simulink model "Grid_Forming_Droop_Control"  (R2022b)
settings: Solver=VariableStepAuto  StartTime=0.0  StopTime=50  RelTol=1e-3
values from neighbouring files (symbols this model uses):
  C_dc = 0.008*(n)    (= 1.6)    [Grid_Forming_Droop_Control_Code.m]
  C_f = n*300*10^-6    (= 0.06)    [Grid_Forming_Droop_Control_Code.m]
  f_0 = 50    [Grid_Forming_Droop_Control_Code.m]
  i_ll = 5*-1.15*(S_b/Vdc_n)-i_loss_dc    [Grid_Forming_Droop_Control_Code.m]
  i_ul = 5*1.15*(S_b/Vdc_n)+i_loss_dc    [Grid_Forming_Droop_Control_Code.m]
  k_dc = eta_1/(Vdc_n*m_p)    [Grid_Forming_Droop_Control_Code.m]
  K_p = (1/Vdc_n)    [Grid_Forming_Droop_Control_Code.m]
  K_r = 1/R_dc    [Grid_Forming_Droop_Control_Code.m]
  Kff_i = 1    [Grid_Forming_Droop_Control_Code.m]
  Kff_v = 1    [Grid_Forming_Droop_Control_Code.m]
  Ki_i = (1/n)*1.19    (= 0.00595)    [Grid_Forming_Droop_Control_Code.m]
  Ki_v = (n)*1.161022    (= 232.2044)    [Grid_Forming_Droop_Control_Code.m]
  ki_v_ac = 2*0.25    (= 0.5)    [Grid_Forming_Droop_Control_Code.m]
  Kp_i = 0.738891    [Grid_Forming_Droop_Control_Code.m]
  Kp_v = 0.52    [Grid_Forming_Droop_Control_Code.m]
  kp_v_ac = 0.001    [Grid_Forming_Droop_Control_Code.m]
  L_f = (1/n)*200*10^-6    (= 1e-06)    [Grid_Forming_Droop_Control_Code.m]
  m_p = (2*pi*(f_0*0.01))/(S_b)    [Grid_Forming_Droop_Control_Code.m]
  n = 200    [Grid_Forming_Droop_Control_Code.m]
  R_dc = (Vdc_n/(0.05*(S_b)/Vdc_n))    [Grid_Forming_Droop_Control_Code.m]
  R_f = 0.001/n    (= 5e-06)    [Grid_Forming_Droop_Control_Code.m]
  S_b = 10*(10^6)    (= 10000000)    [Grid_Forming_Droop_Control_Code.m]
  T_en = T_load-0.5    (= 24.5)    [Grid_Forming_Droop_Control_Code.m]
  T_s = 1e-4    (= 0.0001)    [Grid_Forming_Droop_Control_Code.m]
  tau_dc = 0.05    [Grid_Forming_Droop_Control_Code.m]
  V_m = sqrt(2/3)*V1_rms    [Grid_Forming_Droop_Control_Code.m]
  Vdc_n = 3*V_m    [Grid_Forming_Droop_Control_Code.m]
  Vg = 1000    [Grid_Forming_Droop_Control_Code.m]
  w_b = 2*pi*f_b    (= 314.159265359)    [Grid_Forming_Droop_Control_Code.m]
  w_f = 2*pi*0.1*f_b    (= 31.4159265359)    [Grid_Forming_Droop_Control_Code.m]
undefined symbols (not defined in the file or in its folder): i_dc
libraries: spsSeriesRLCBranchLib x8, spsVoltageMeasurementLib x8, spsCurrentMeasurementLib x7, spsabctodq0Lib x7, spsGroundLib x3, spsFirstOrderFilterLib x2, cstblocks x1, spsControlledCurrentSourceLib x1, slpidlib x1, spsThreePhaseSourceLib x1, spsUniversalBridgeLib x1, spsdq0toabcLib x1
settings Model: Creator=alper.cakiroglu  LastModifiedBy=alper.cakiroglu

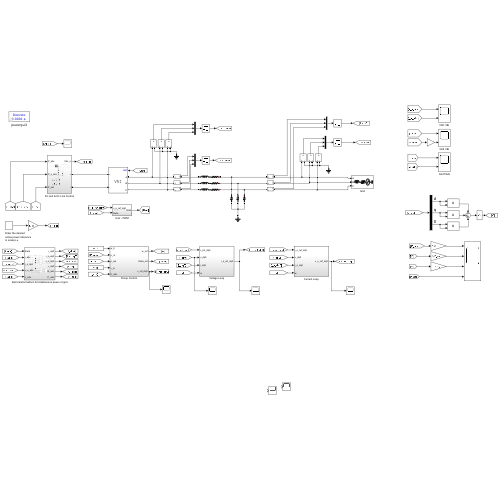
[thumbnail: Simulink's stored preview of the top-level diagram]
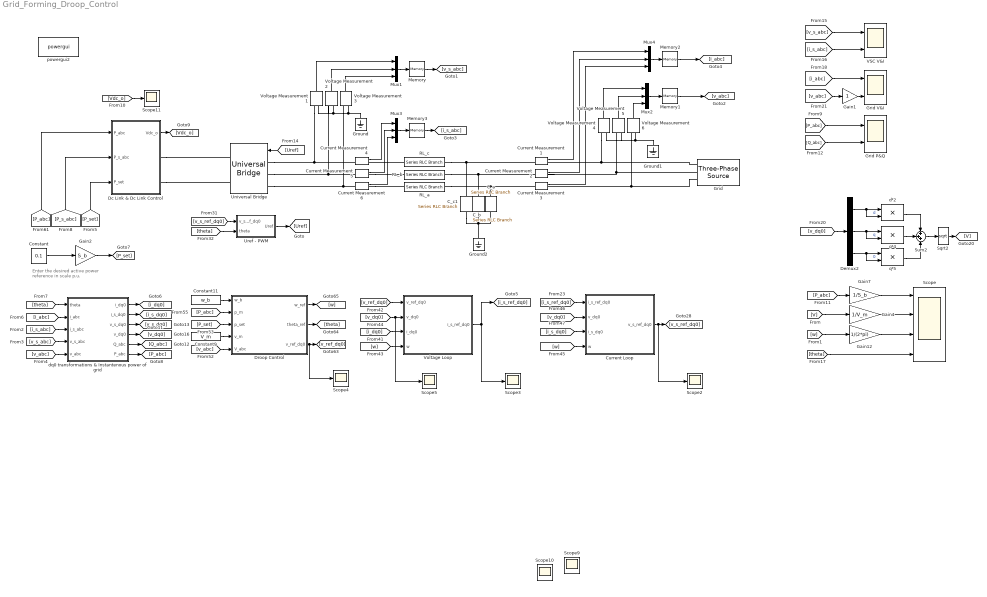
== system Grid_Forming_Droop_Control ==
  note: Enter the desired active power reference
      | in scale p.u.
  C_a : spsSeriesRLCBranchLib/Series RLC Branch  LConnTagsString=__new0  RConnTagsString=__new0  BranchType=C  Resistance=1  Inductance=1e-3  SetiL0=off  InitialCurrent=0  Capacitance=C_f  Setx0=off  InitialVoltage=165  Measurements=None
  C_b : spsSeriesRLCBranchLib/Series RLC Branch  LConnTagsString=__new0  RConnTagsString=__new0  BranchType=C  Resistance=1  Inductance=1e-3  SetiL0=off  InitialCurrent=0  Capacitance=C_f  Setx0=off  InitialVoltage=165  Measurements=None
  C_c1 : spsSeriesRLCBranchLib/Series RLC Branch  LConnTagsString=__new0  RConnTagsString=__new0  BranchType=C  Resistance=1  Inductance=1e-3  SetiL0=off  InitialCurrent=0  Capacitance=C_f  Setx0=off  InitialVoltage=165  Measurements=None
  Constant : Constant  Value=0.1
  Constant11 : Constant  Value=w_b
  Constant9 : Constant  Value=V_m
  Current Loop : Subsystem
  Current Measurement{1..6} (6 alike) : spsCurrentMeasurementLib/Current Measurement  PhasorSimulation=off  OutputType=Complex  PSBequivalent=0
  Dc Link & Dc Link Control : Subsystem
  Demux2 : Demux  Outputs=3
  Droop Control : Subsystem
  Gain1 : Gain
  Gain12 : Gain  Gain=1/(2*pi)
  Gain2 : Gain  Gain=S_b
  Gain4 : Gain  Gain=1/V_m
  Gain7 : Gain  Gain=1/S_b
  Grid : spsThreePhaseSourceLib/Three-Phase Source  InternalConnection=Yg  VoltagePhases=off  Voltage=Vg  PhaseAngle=0  Voltage_phases=[25e3 25e3 25e3]/sqrt(3)  PhaseAngles_phases=[0 -120 +120]  Frequency=f_0  NonIdealSource=on  SpecifyImpedance=on  Resistance=0.8929  Inductance=16.58e-3  ShortCircuitLevel=S_b  BaseVoltage=Vg  XRratio=10  BusType=swing  Pref=10e3  Qref=0  Prefabc=[10e3, 10e3, 10e3]  Qrefabc=[0, 0, 0]  Qmin=-inf  Qmax=inf
  Grid P&Q : Scope  NumInputPorts=2
  Grid V&I : Scope  NumInputPorts=2
  Ground : spsGroundLib/Ground  LConnTagsString=a
  Ground1 : spsGroundLib/Ground  LConnTagsString=a
  Ground2 : spsGroundLib/Ground  LConnTagsString=a
  Memory{,1..3} (4 alike) : Memory
  Mux{1..4} (4 alike) : Mux  Inputs=3
  RL_a : spsSeriesRLCBranchLib/Series RLC Branch  LConnTagsString=__new0  RConnTagsString=__new0  BranchType=RL  Resistance=R_f  Inductance=L_f  SetiL0=off  InitialCurrent=0  Capacitance=1e-6  Setx0=off  InitialVoltage=0  Measurements=Branch voltage and current
  RL_b : spsSeriesRLCBranchLib/Series RLC Branch  LConnTagsString=__new0  RConnTagsString=__new0  BranchType=RL  Resistance=R_f  Inductance=L_f  SetiL0=off  InitialCurrent=0  Capacitance=1e-6  Setx0=off  InitialVoltage=0  Measurements=None
  RL_c : spsSeriesRLCBranchLib/Series RLC Branch  LConnTagsString=__new0  RConnTagsString=__new0  BranchType=RL  Resistance=R_f  Inductance=L_f  SetiL0=off  InitialCurrent=0  Capacitance=1e-6  Setx0=off  InitialVoltage=0  Measurements=None
  Scope : Scope  NumInputPorts=4
  Scope{2..5,9..11} (7 alike) : Scope
  Sqrt2 : Sqrt
  Sum2 : Sum  Inputs=+++  InputSameDT=on  SaturateOnIntegerOverflow=on  OutDataTypeStr=Inherit: Same as first input
  Universal Bridge : spsUniversalBridgeLib/Universal Bridge  Arms=3  SnubberResistance=1e5  SnubberCapacitance=inf  Device=Average-model based VSC  Ron=1e-3  Lon=0  ForwardVoltages="[  0  0  ]"  ForwardVoltage=0  GTOparameters=[ 10e-6 , 20e-6 ]  IGBTparameters=[ 1e-6 , 2e-6 ]  Measurements=None  Measurements_2=None  converterType=Rectifier
  Uref - PWM : Subsystem
  VSC V&I : Scope  NumInputPorts=2
  Voltage Loop : Subsystem
  Voltage Measurement{1..6} (6 alike) : spsVoltageMeasurementLib/Voltage Measurement  PhasorSimulation=off  OutputType=Complex  PSBequivalent=0
  dq0 transformations & Instantenous power of grid : Subsystem
  d²2 : Product  InputSameDT=on  RndMeth=Zero  SaturateOnIntegerOverflow=on  OutDataTypeStr=Inherit: Same as first input
  powergui2 : sps_lib/powergui  Priority=1  SimulationMode=Discrete  SampleTime=T_s  frequency=50  Iterations=50  frequencyindice=0  Pbase=100e6  ErrMax=0.0001  UnitsV=kV  UnitsW=MW  buscounter=0  FunctionMessages=off  echomessages=off  EnableUseOfTLC=off  CurrentSourceSwitches=off  DisableSnubberDevices=off  DisableRonSwitches=off  DisableVfSwitches=off  DisplayEquations=off  AutomaticDiscreteSolvers=off  SolverType=Tustin/Backward Euler (TBE)  Interpol=off  ExternalGateDelay=off  methode=off  Ts=100  x0status=blocks  SPID=off  SwTol=0  HookPort=off  NonlinearTolerance=1e-4  nMaxIteration=100  ContinueOnMaxIteration=off  RestoreLinks=warning  ResistiveCurrentMeasurement=off  Frange=[0:2:500]  Ylog=off  Xlog=on  ShowGrid=off  save=off  variable=ZData  structure=0  ZoomFFT=off  StartTime=0.0  cycles=1  DisplayStyle=1  fundamental=60  FreqAxis=off  MaxFrequency=1000  frequencyindicesteady=1  RmsSteady=1  display=off
  q²4 : Product  InputSameDT=on  RndMeth=Zero  SaturateOnIntegerOverflow=on  OutDataTypeStr=Inherit: Same as first input
  q²5 : Product  InputSameDT=on  RndMeth=Zero  SaturateOnIntegerOverflow=on  OutDataTypeStr=Inherit: Same as first input
  wires:
  Voltage Measurement2/1 -> Mux1/2
  Voltage Measurement1/1 -> Mux1/1
  Voltage Measurement3/1 -> Mux1/3
  Memory/1 -> [v_s_abc]
  Mux1/1 -> Memory/1
  Memory1/1 -> [v_abc]
  Voltage Measurement6/1 -> Mux2/3
  Voltage Measurement4/1 -> Mux2/1
  Voltage Measurement5/1 -> Mux2/2
  Mux2/1 -> Memory1/1
  Mux3/1 -> Memory3/1
  Memory3/1 -> [i_s_abc]
  Current Measurement4/1 -> Mux3/1
  Current Measurement5/1 -> Mux3/2
  Current Measurement6/1 -> Mux3/3
  Memory2/1 -> [i_abc]
  Mux4/1 -> Memory2/1
  Current Measurement1/1 -> Mux4/1
  Current Measurement2/1 -> Mux4/2
  Current Measurement3/1 -> Mux4/3
  [v_dq0] -> Demux2/1
  Gain12/1 -> Scope/3
  [P_abc] -> Gain7/1
  Demux2/3 -> q²5/1, q²5/2  "0"
  Demux2/2 -> q²4/1, q²4/2  "q"
  q²5/1 -> Sum2/3
  Sum2/1 -> Sqrt2/1
  d²2/1 -> Sum2/1
  Constant/1 -> Gain2/1
  Sqrt2/1 -> [V]
  Demux2/1 -> d²2/1, d²2/2  "d"
  [w] -> Gain12/1
  [theta] -> Scope/4
  Gain4/1 -> Scope/2
  q²4/1 -> Sum2/2
  Gain2/1 -> [P_set]
  Gain7/1 -> Scope/1
  [V] -> Gain4/1
  [w] -> Voltage Loop/4(w)
  Droop Control/3(v_ref_dq0) -> Scope4/1, [v_ref_dq0]
  [v_dq0] -> Current Loop/2(v_dq0)
  Droop Control/1(w_ref) -> [w]
  Current Loop/1(v_s_ref_dq0) -> Scope2/1, [v_s_ref_dq0]
  Constant11/1 -> Droop Control/1(w_b)
  Voltage Loop/1(i_s_ref_dq0) -> Scope3/1, [i_s_ref_dq0]
  [w] -> Current Loop/4(w)
  [v_abc] -> Droop Control/5(V_abc)
  [v_ref_dq0] -> Voltage Loop/1(v_ref_dq0)
  [i_dq0] -> Voltage Loop/3(i_dq0)
  [i_s_dq0] -> Current Loop/3(i_s_dq0)
  [v_dq0] -> Scope5/1, Voltage Loop/2(v_dq0)
  Droop Control/2(theta_ref) -> [theta]
  [P_set] -> Droop Control/3(p_set)
  [P_abc] -> Droop Control/2(p_m)
  [Vdc_o] -> Scope11/1
  Constant9/1 -> Droop Control/4(v_m)
  Dc Link & Dc Link Control/1(Vdc_o) -> [Vdc_o]
  [P_abc] -> Dc Link & Dc Link Control/1(P_abc)
  [P_s_abc] -> Dc Link & Dc Link Control/2(P_s_abc)
  [P_set] -> Dc Link & Dc Link Control/3(P_set)
  [Uref] -> Universal Bridge/1
  [v_s_abc] -> VSC V&I/1
  [i_s_abc] -> VSC V&I/2
  Uref - PWM/1(Uref) -> [Uref]
  [v_s_ref_dq0] -> Uref - PWM/1(v_s_ref_dq0)
  [theta] -> Uref - PWM/2(theta)
  [i_abc] -> Grid V&I/1
  [v_abc] -> Gain1/1
  Gain1/1 -> Grid V&I/2
  [i_abc] -> dq0 transformations & Instantenous power of grid/2(i_abc)
  [i_s_abc] -> dq0 transformations & Instantenous power of grid/3(i_s_abc)
  [v_s_abc] -> dq0 transformations & Instantenous power of grid/4(v_s_abc)
  [v_abc] -> dq0 transformations & Instantenous power of grid/5(v_abc)
  dq0 transformations & Instantenous power of grid/1(i_dq0) -> [i_dq0]
  dq0 transformations & Instantenous power of grid/2(i_s_dq0) -> [i_s_dq0]
  dq0 transformations & Instantenous power of grid/3(v_s_dq0) -> [v_s_dq0]
  dq0 transformations & Instantenous power of grid/4(v_dq0) -> [v_dq0]
  dq0 transformations & Instantenous power of grid/5(Q_abc) -> [Q_abc]
  dq0 transformations & Instantenous power of grid/6(P_abc) -> [P_abc]
  [theta] -> dq0 transformations & Instantenous power of grid/1(theta)
  [i_s_ref_dq0] -> Current Loop/1(i_s_ref_dq0)
  [Q_abc] -> Grid P&Q/2
  [P_abc] -> Grid P&Q/1
  connections:
  Universal Bridge/LConn1 -- Voltage Measurement1/LConn1 -- Current Measurement4/LConn1
  Universal Bridge/LConn2 -- Voltage Measurement2/LConn1 -- Current Measurement5/LConn1
  Universal Bridge/LConn3 -- Voltage Measurement3/LConn1 -- Current Measurement6/LConn1
  Voltage Measurement1/LConn2 -- Voltage Measurement2/LConn2 -- Voltage Measurement3/LConn2 -- Ground/LConn1
  RL_c/RConn1 -- Current Measurement4/RConn1
  Current Measurement5/RConn1 -- RL_b/RConn1
  Current Measurement6/RConn1 -- RL_a/RConn1
  Ground2/LConn1 -- C_c1/RConn1 -- C_a/RConn1 -- C_b/RConn1
  RL_c/LConn1 -- C_c1/LConn1 -- Current Measurement1/LConn1
  RL_b/LConn1 -- C_b/LConn1 -- Current Measurement2/LConn1
  RL_a/LConn1 -- C_a/LConn1 -- Current Measurement3/LConn1
  Grid/RConn1 -- Voltage Measurement4/LConn1 -- Current Measurement1/RConn1
  Current Measurement2/RConn1 -- Voltage Measurement5/LConn1 -- Grid/RConn2
  Grid/RConn3 -- Voltage Measurement6/LConn1 -- Current Measurement3/RConn1
  Voltage Measurement6/LConn2 -- Voltage Measurement4/LConn2 -- Voltage Measurement5/LConn2 -- Ground1/LConn1
  Dc Link & Dc Link Control/RConn2 -- Universal Bridge/RConn2
  Dc Link & Dc Link Control/RConn1 -- Universal Bridge/RConn1

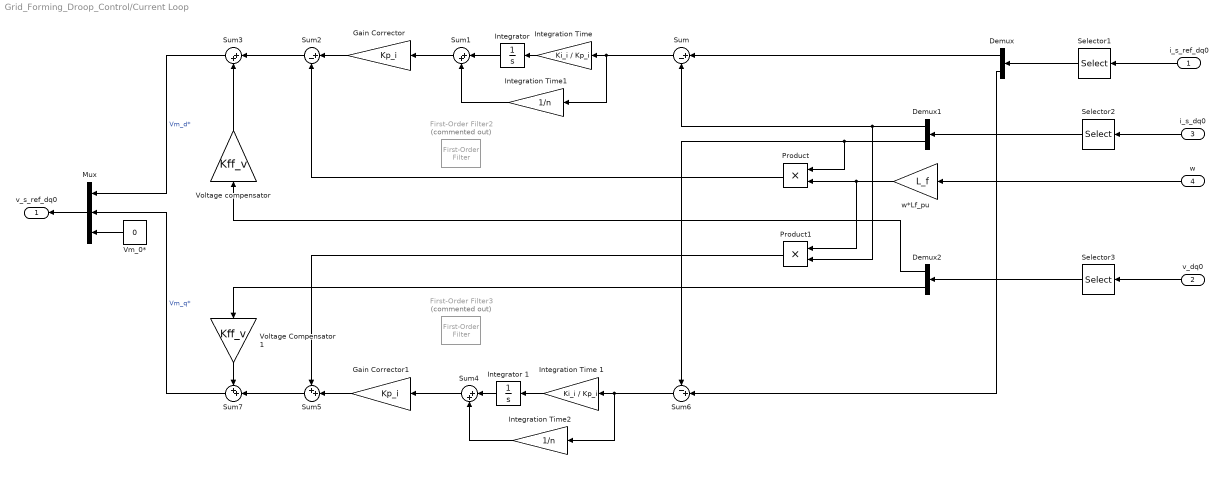
== system Grid_Forming_Droop_Control/Current Loop ==
  i_s_ref_dq0 : Inport
  v_dq0 : Inport  Port=2
  i_s_dq0 : Inport  Port=3
  w : Inport  Port=4
  Demux : Demux  Outputs=2
  Demux1 : Demux  Outputs=2
  Demux2 : Demux  Outputs=2
  First-Order Filter2 : spsFirstOrderFilterLib/First-Order Filter  Commented=on  FilterType=Lowpass  Tc=25e-3  Ts=0  Initialize=on  Vac_Init=[0, 0, 50]  Vdc_Init=1  PlotResponse=off  FreqRange="[0,  200,  1]"
  First-Order Filter3 : spsFirstOrderFilterLib/First-Order Filter  Commented=on  FilterType=Lowpass  Tc=25e-3  Ts=0  Initialize=on  Vac_Init=[0, 0, 50]  Vdc_Init=0  PlotResponse=off  FreqRange="[0,  200,  1]"
  Gain Corrector : Gain  Gain=Kp_i
  Gain Corrector1 : Gain  Gain=Kp_i
  Integration Time : Gain  Gain=Ki_i / Kp_i
  Integration Time 1 : Gain  Gain=Ki_i / Kp_i
  Integration Time1 : Gain  Gain=1/n
  Integration Time2 : Gain  Gain=1/n
  Integrator : Integrator  InitialCondition=0.0001
  Integrator 1 : Integrator
  Mux : Mux  Inputs=3
  Product : Product  RndMeth=Zero
  Product1 : Product  RndMeth=Zero
  Selector1 : Selector  InputPortWidth=3  IndexOptions=Index vector (dialog)  Indices=[1 2]  OutputSizes=1
  Selector2 : Selector  InputPortWidth=3  IndexOptions=Index vector (dialog)  Indices=[1 2]  OutputSizes=1
  Selector3 : Selector  InputPortWidth=3  IndexOptions=Index vector (dialog)  Indices=[1 2]  OutputSizes=1
  Sum : Sum  Inputs=|+-
  Sum1 : Sum  Inputs=|++
  Sum2 : Sum  Inputs=|+-
  Sum3 : Sum  Inputs=|++
  Sum4 : Sum  Inputs=|++
  Sum5 : Sum  Inputs=++|
  Sum6 : Sum  Inputs=-+|
  Sum7 : Sum  Inputs=++|
  Vm_0* : Constant  Value=0
  Voltage Compensator 1 : Gain  Gain=Kff_v
  Voltage compensator : Gain  Gain=Kff_v
  w*Lf_pu : Gain  Gain=L_f
  v_s_ref_dq0 : Outport  VectorParamsAs1DForOutWhenUnconnected=off
  wires:
  Sum/1 -> Integration Time/1, Integration Time1/1
  Integration Time 1/1 -> Integrator 1/1
  Integration Time/1 -> Integrator/1
  Sum5/1 -> Sum7/2
  Sum6/1 -> Integration Time 1/1, Integration Time2/1
  Demux/1 -> Sum/1
  Sum3/1 -> Mux/1  "Vm_d*"
  Sum7/1 -> Mux/2  "Vm_q*"
  Demux2/2 -> Voltage Compensator 1/1
  Voltage Compensator 1/1 -> Sum7/1
  Product/1 -> Sum2/2
  w*Lf_pu/1 -> Product1/1, Product/2
  i_s_ref_dq0/1 -> Selector1/1
  v_dq0/1 -> Selector3/1
  Integrator 1/1 -> Sum4/1
  Voltage compensator/1 -> Sum3/2
  Sum1/1 -> Gain Corrector/1
  Sum2/1 -> Sum3/1
  Sum4/1 -> Gain Corrector1/1
  Demux/2 -> Sum6/2
  Selector1/1 -> Demux/1
  Gain Corrector/1 -> Sum2/1
  w/1 -> w*Lf_pu/1
  Mux/1 -> v_s_ref_dq0/1
  Selector2/1 -> Demux1/1
  i_s_dq0/1 -> Selector2/1
  Selector3/1 -> Demux2/1
  Demux1/2 -> Product/1, Sum6/1
  Vm_0*/1 -> Mux/3
  Integrator/1 -> Sum1/1
  Demux1/1 -> Product1/2, Sum/2
  Demux2/1 -> Voltage compensator/1
  Product1/1 -> Sum5/1
  Gain Corrector1/1 -> Sum5/2
  Integration Time1/1 -> Sum1/2
  Integration Time2/1 -> Sum4/2

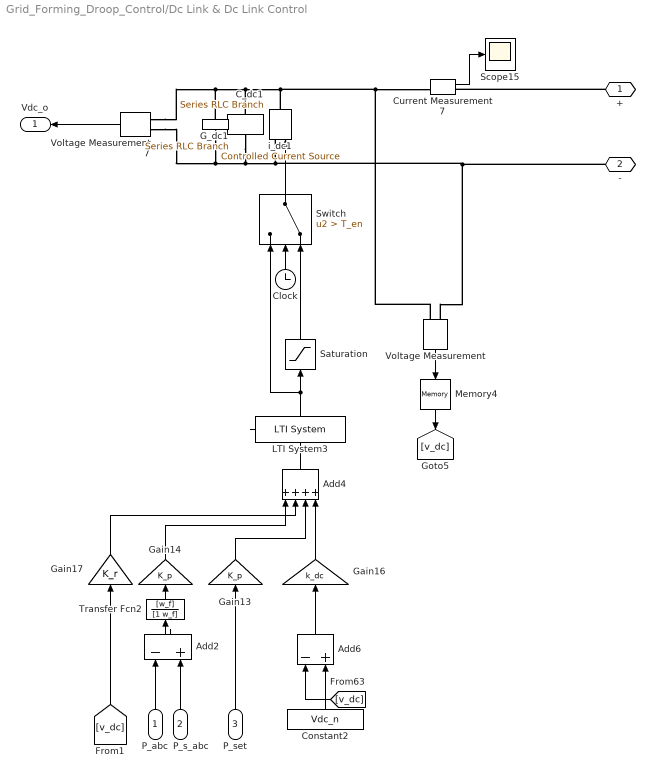
== system Grid_Forming_Droop_Control/Dc Link & Dc Link Control ==
  P_abc : Inport
  P_s_abc : Inport  Port=2
  P_set : Inport  Port=3
  Add2 : Sum  Inputs=+-
  Add4 : Sum  Inputs=++++
  Add6 : Sum  Inputs=+-
  C_dc1 : spsSeriesRLCBranchLib/Series RLC Branch  LConnTagsString=__new0  RConnTagsString=__new0  BranchType=C  Resistance=1  Inductance=1e-3  SetiL0=off  InitialCurrent=0  Capacitance=C_dc  Setx0=off  InitialVoltage=Vdc_n  Measurements=None
  Clock : Clock
  Constant2 : Constant  Value=Vdc_n
  Current Measurement7 : spsCurrentMeasurementLib/Current Measurement  PhasorSimulation=off  OutputType=Complex  PSBequivalent=0
  G_dc1 : spsSeriesRLCBranchLib/Series RLC Branch  LConnTagsString=__new0  RConnTagsString=__new0  BranchType=R  Resistance=R_dc  Inductance=1e-3  SetiL0=off  InitialCurrent=0  Capacitance=1e-6  Setx0=off  InitialVoltage=0  Measurements=None
  Gain13 : Gain  Gain=K_p
  Gain14 : Gain  Gain=K_p
  Gain16 : Gain  Gain=k_dc
  Gain17 : Gain  Gain=K_r
  LTI System3 : cstblocks/LTI System  sys=tf(1,[tau_dc 1])  IC=[]
  Memory4 : Memory
  Saturation : Saturate  UpperLimit=i_ul  LowerLimit=i_ll
  Scope15 : Scope
  Switch : Switch  Criteria=u2 > Threshold  Threshold=T_en  SaturateOnIntegerOverflow=off  InputSameDT=off
  Transfer Fcn2 : TransferFcn  Numerator=[w_f]  Denominator=[1 w_f]
  Voltage Measurement : spsVoltageMeasurementLib/Voltage Measurement  PhasorSimulation=off  OutputType=Complex  PSBequivalent=0
  Voltage Measurement7 : spsVoltageMeasurementLib/Voltage Measurement  PhasorSimulation=off  OutputType=Complex  PSBequivalent=0
  i_dc1 : spsControlledCurrentSourceLib/Controlled Current Source  Initialize=off  Source_Type=DC  Amplitude=i_dc  Phase=0  Frequency=0  Measurements=None
  + : PMIOPort  Side=Right
  - : PMIOPort  Port=2  Side=Right
  Vdc_o : Outport
  wires:
  Clock/1 -> Switch/2
  Add2/1 -> Transfer Fcn2/1
  Gain16/1 -> Add4/1
  Current Measurement7/1 -> Scope15/1
  Switch/1 -> i_dc1/1
  Saturation/1 -> Switch/1
  Transfer Fcn2/1 -> Gain14/1
  Gain17/1 -> Add4/3
  Voltage Measurement/1 -> Memory4/1
  Add6/1 -> Gain16/1
  LTI System3/1 -> Switch/3, Saturation/1
  Memory4/1 -> [v_dc]
  Gain14/1 -> Add4/4
  Constant2/1 -> Add6/1
  [v_dc] -> Add6/2
  Add4/1 -> LTI System3/1
  P_s_abc/1 -> Add2/1
  Gain13/1 -> Add4/2
  P_set/1 -> Gain13/1
  Voltage Measurement7/1 -> Vdc_o/1
  P_abc/1 -> Add2/2
  [v_dc] -> Gain17/1
  connections:
  +/RConn1 -- Current Measurement7/RConn1
  Voltage Measurement/LConn1 -- Current Measurement7/LConn1 -- G_dc1/LConn1 -- Voltage Measurement7/LConn1 -- C_dc1/LConn1 -- i_dc1/RConn1
  i_dc1/LConn1 -- -/RConn1 -- Voltage Measurement/LConn2 -- G_dc1/RConn1 -- Voltage Measurement7/LConn2 -- C_dc1/RConn1

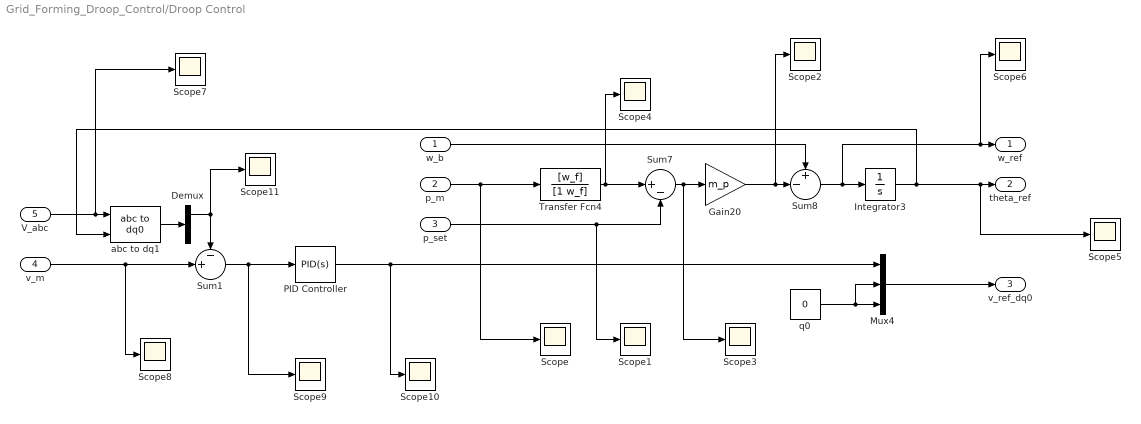
== system Grid_Forming_Droop_Control/Droop Control ==
  w_b : Inport
  p_m : Inport  Port=2
  p_set : Inport  Port=3
  v_m : Inport  Port=4
  V_abc : Inport  Port=5
  Demux : Demux  Outputs=3
  Gain20 : Gain  Gain=m_p
  Integrator3 : Integrator
  Mux4 : Mux  Inputs=3
  PID Controller : slpidlib/PID Controller  Controller=PID  Form=Parallel  TimeDomain=Continuous-time  UseExternalTs=off  SampleTime=-1  IntegratorMethod=Forward Euler  FilterMethod=Forward Euler  ControllerParametersSource=internal  P=kp_v_ac  I=ki_v_ac  UseKiTs=off  D=0  N=100  UseFilter=on  TunerSelectOption=Transfer Function Based (PID Tuner App)  InitialConditionSource=internal  InitialConditionForIntegrator=0  InitialConditionForFilter=0  DifferentiatorICPrevScaledInput=0  ExternalReset=none  TrackingMode=off  Kt=1  LimitOutput=off  SatLimitsSource=internal  UpperSaturationLimit=inf  LowerSaturationLimit=-inf  LinearizeAsGain=on  AntiWindupMode=none  Kb=1  LimitIntegrator=off  UpperIntegratorSaturationLimit=inf  LowerIntegratorSaturationLimit=-inf  POutMin=[]  POutMax=[]  IOutMin=[]  IOutMax=[]  DOutMin=[]  DOutMax=[]  NOutMin=[]  NOutMax=[]  SumOutMin=[]  SumOutMax=[]  SaturationOutMin=[]  SaturationOutMax=[]  PParamMin=[]  PParamMax=[]  IParamMin=[]  IParamMax=[]  DParamMin=[]  DParamMax=[]  NParamMin=[]  NParamMax=[]  KbParamMin=[]  KbParamMax=[]  KtParamMin=[]  KtParamMax=[]  KbOutMin=[]  KbOutMax=[]  KtOutMin=[]  KtOutMax=[]  IntegratorOutMin=[]  IntegratorOutMax=[]  FilterOutMin=[]  FilterOutMax=[]  SumI1OutMin=[]  SumI1OutMax=[]  SumI2OutMin=[]  SumI2OutMax=[]  SumI3OutMin=[]  SumI3OutMax=[]  SumI4OutMin=[]  SumI4OutMax=[]  SumDOutMin=[]  SumDOutMax=[]  DifferentiatorOutMin=[]  DifferentiatorOutMax=[]  FilterDiffOutCoefMin=[]  FilterDiffOutCoefMax=[]  ReciprocalOutMin=[]  ReciprocalOutMax=[]  SumDenOutMin=[]  SumDenOutMax=[]  SumNumOutMin=[]  SumNumOutMax=[]  DivideOutMin=[]  DivideOutMax=[]  UdiffTsProdOutMin=[]  UdiffTsProdOutMax=[]  NTsProdOutMin=[]  NTsProdOutMax=[]  UintegralTsProdOutMin=[]  UintegralTsProdOutMax=[]  UngainTsProdOutMin=[]  UngainTsProdOutMax=[]  ClampingZeroOutDataTypeStr=Inherit: Inherit via back propagation  ClampingZeroOutMin=[]  ClampingZeroOutMax=[]  FilterDenConstantOutDataTypeStr=Inherit: Inherit via back propagation  FilterDenConstantOutMin=[]  FilterDenConstantOutMax=[]  PCopyOutDataTypeStr=Inherit: Inherit via back propagation  PCopyOutMin=[]  PCopyOutMax=[]  NCopyOutDataTypeStr=Inherit: Inherit via back propagation  NCopyOutMin=[]  NCopyOutMax=[]  IntegratorContinuousStateAttributes=''  IntegratorStateMustResolveToSignalObject=off  IntegratorRTWStateStorageClass=Auto  FilterContinuousStateAttributes=''  FilterStateMustResolveToSignalObject=off  FilterRTWStateStorageClass=Auto  ParallelPVariant=InternalParameters  IdealPVariant=Disabled  IVariant=InternalParameters  DVariant=InternalParameters  IntegratorVariant=Continuous  SatVariant=Disabled  AWVariant=Passthrough  PCopyVariant=Disabled  TRVariant=Disabled  FdbkBlocksVariant=Forward  IdealPFdbkVariant=Disabled  SatFdbkVariant=Disabled  DerivativeFilterVariant=ContFilter  NVariant=InternalParameters  NCopyVariant=Disabled  FilterICVariant=InternalICsFilter  IntegratorICVariant=InternalICs  ExternalResetVariant=Disabled  TRSumVariant=Passthrough  SumFdbkVariant=Disabled  SumVariant=Sum_PID  TsampFilterVariant=InternalTs  TsampNgainVariant=Passthrough  TsampIntegralVariant=Passthrough  ExternalSaturationOutDataTypeStr=Inherit: Same as second input
  Scope{,1..11} (12 alike) : Scope
  Sum1 : Sum  Inputs=-+|
  Sum7 : Sum  Inputs=|+-
  Sum8 : Sum  Inputs=+-|
  Transfer Fcn4 : TransferFcn  Numerator=[w_f]  Denominator=[1 w_f]
  abc to dq1 : spsabctodq0Lib/abc to dq0  Alignment=90 degrees behind phase A axis
  q0 : Constant  Value=0
  w_ref : Outport  VectorParamsAs1DForOutWhenUnconnected=off
  theta_ref : Outport  Port=2  VectorParamsAs1DForOutWhenUnconnected=off
  v_ref_dq0 : Outport  Port=3  VectorParamsAs1DForOutWhenUnconnected=off
  wires:
  Demux/1 -> Scope11/1, Sum1/1
  abc to dq1/1 -> Demux/1
  Transfer Fcn4/1 -> Scope4/1, Sum7/1
  Mux4/1 -> v_ref_dq0/1
  q0/1 -> Mux4/3, Mux4/2
  Sum8/1 -> Integrator3/1, Scope6/1, w_ref/1
  Gain20/1 -> Scope2/1, Sum8/2
  Sum7/1 -> Scope3/1, Gain20/1
  p_m/1 -> Transfer Fcn4/1, Scope/1
  p_set/1 -> Sum7/2, Scope1/1
  w_b/1 -> Sum8/1
  V_abc/1 -> Scope7/1, abc to dq1/1
  Sum1/1 -> PID Controller/1, Scope9/1
  v_m/1 -> Scope8/1, Sum1/2
  Integrator3/1 -> abc to dq1/2, Scope5/1, theta_ref/1
  PID Controller/1 -> Scope10/1, Mux4/1

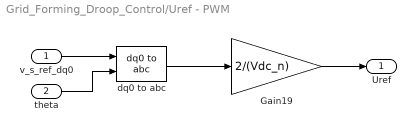
== system Grid_Forming_Droop_Control/Uref - PWM ==
  v_s_ref_dq0 : Inport
  theta : Inport  Port=2
  Gain19 : Gain  Gain=2/(Vdc_n)
  dq0 to abc : spsdq0toabcLib/dq0 to abc  Alignment=90 degrees behind phase A axis
  Uref : Outport
  wires:
  v_s_ref_dq0/1 -> dq0 to abc/1
  theta/1 -> dq0 to abc/2
  dq0 to abc/1 -> Gain19/1
  Gain19/1 -> Uref/1

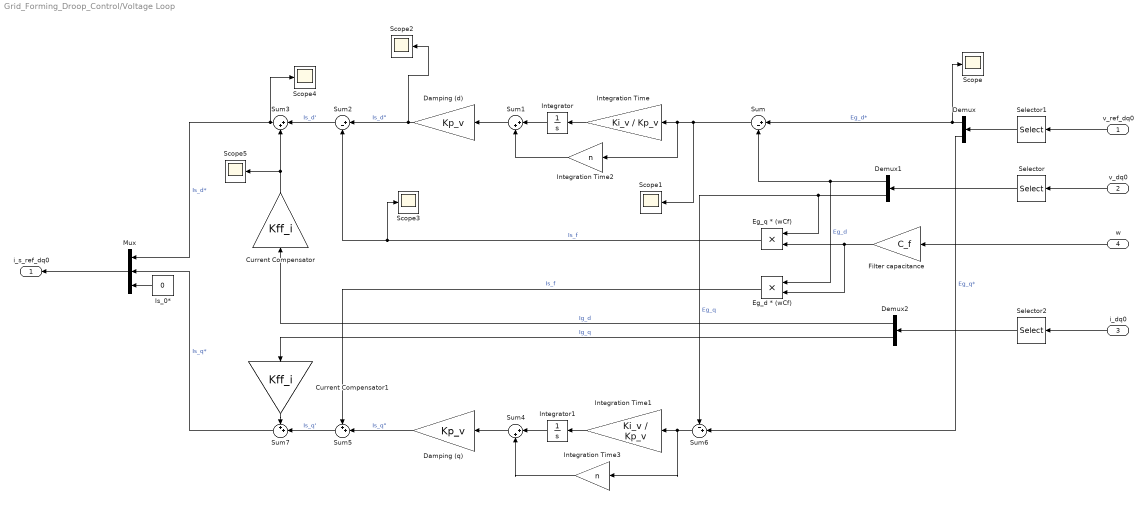
== system Grid_Forming_Droop_Control/Voltage Loop ==
  v_ref_dq0 : Inport
  v_dq0 : Inport  Port=2
  i_dq0 : Inport  Port=3
  w : Inport  Port=4
  Current Compensator : Gain  Gain=Kff_i
  Current Compensator1 : Gain  Gain=Kff_i
  Damping (d) : Gain  Gain=Kp_v
  Damping (q) : Gain  Gain=Kp_v
  Demux : Demux  Outputs=2
  Demux1 : Demux  Outputs=2
  Demux2 : Demux  Outputs=2
  Eg_d * (wCf) : Product  RndMeth=Zero
  "Eg_q * (wCf) " : Product  RndMeth=Zero
  Filter capacitance : Gain  Gain=C_f
  Integration Time : Gain  Gain=Ki_v / Kp_v
  Integration Time1 : Gain  Gain=Ki_v / Kp_v
  Integration Time2 : Gain  Gain=n
  Integration Time3 : Gain  Gain=n
  Integrator : Integrator
  Integrator1 : Integrator
  Is_0* : Constant  Value=0
  Mux : Mux  Inputs=3
  Scope{,1..5} (6 alike) : Scope
  Selector : Selector  InputPortWidth=3  IndexOptions=Index vector (dialog)  Indices=[1 2]  OutputSizes=1
  Selector1 : Selector  InputPortWidth=3  IndexOptions=Index vector (dialog)  Indices=[1 2]  OutputSizes=1
  Selector2 : Selector  InputPortWidth=3  IndexOptions=Index vector (dialog)  Indices=[1 2]  OutputSizes=1
  Sum : Sum  Inputs=|+-
  Sum1 : Sum  Inputs=|++
  Sum2 : Sum  Inputs=|+-
  Sum3 : Sum  Inputs=|++
  Sum4 : Sum  Inputs=|++
  Sum5 : Sum  Inputs=++|
  Sum6 : Sum  Inputs=-+|
  Sum7 : Sum  Inputs=++|
  i_s_ref_dq0 : Outport  VectorParamsAs1DForOutWhenUnconnected=off
  wires:
  Is_0*/1 -> Mux/3
  w/1 -> Filter capacitance/1
  Integration Time1/1 -> Integrator1/1
  Integrator1/1 -> Sum4/1
  Demux/2 -> Sum6/2  "Eg_q*"
  v_ref_dq0/1 -> Selector1/1
  Eg_d * (wCf)/1 -> Sum5/1  "Is_f"
  Sum7/1 -> Mux/2  "Is_q*"
  Demux2/2 -> Current Compensator1/1  "Ig_q"
  Demux/1 -> Scope/1, Sum/1  "Eg_d*"
  Sum6/1 -> Integration Time3/1, Integration Time1/1
  Demux2/1 -> Current Compensator/1  "Ig_d"
  Sum2/1 -> Sum3/1  "Is_d'"
  Current Compensator/1 -> Scope5/1, Sum3/2
  Demux1/1 -> Eg_d * (wCf)/1, Sum/2  "Eg_d"
  Current Compensator1/1 -> Sum7/1
  "Eg_q * (wCf) "/1 -> Scope3/1, Sum2/2  "Is_f"
  Demux1/2 -> "Eg_q * (wCf) "/1, Sum6/1  "Eg_q"
  Filter capacitance/1 -> "Eg_q * (wCf) "/2, Eg_d * (wCf)/2
  Damping (d)/1 -> Scope2/1, Sum2/1  "Is_d\""
  i_dq0/1 -> Selector2/1
  Sum5/1 -> Sum7/2  "Is_q'"
  Sum1/1 -> Damping (d)/1
  Integrator/1 -> Sum1/1
  Integration Time/1 -> Integrator/1
  Sum4/1 -> Damping (q)/1
  Sum3/1 -> Scope4/1, Mux/1  "Is_d*"
  v_dq0/1 -> Selector/1
  Damping (q)/1 -> Sum5/2  "Is_q\""
  Selector/1 -> Demux1/1
  Selector1/1 -> Demux/1
  Selector2/1 -> Demux2/1
  Mux/1 -> i_s_ref_dq0/1
  Sum/1 -> Scope1/1, Integration Time/1, Integration Time2/1
  Integration Time2/1 -> Sum1/2
  Integration Time3/1 -> Sum4/2

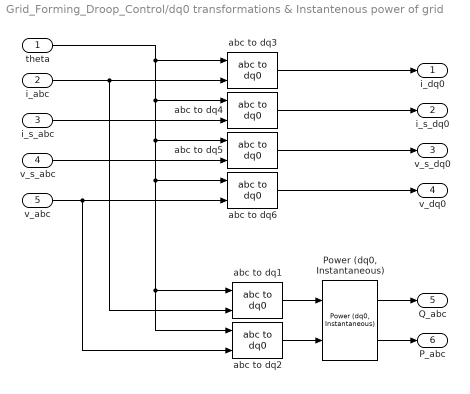
== system Grid_Forming_Droop_Control/dq0 transformations & Instantenous power of grid ==
  theta : Inport
  i_abc : Inport  Port=2
  i_s_abc : Inport  Port=3
  v_s_abc : Inport  Port=4
  v_abc : Inport  Port=5
  "Power (dq0, Instantaneous)" : spsPowerdq0InstantaneousLib/Power (dq0, Instantaneous)
      settings: LibrarySourceBlock=|
      | sps_lib/Sensors and Measurements/Power
      | (dq0, Instantaneous)
  abc to dq{1..6} (6 alike) : spsabctodq0Lib/abc to dq0  Alignment=90 degrees behind phase A axis
  i_dq0 : Outport
  i_s_dq0 : Outport  Port=2
  v_s_dq0 : Outport  Port=3
  v_dq0 : Outport  Port=4
  Q_abc : Outport  Port=5
  P_abc : Outport  Port=6
  wires:
  abc to dq6/1 -> v_dq0/1
  v_abc/1 -> abc to dq2/1, abc to dq6/1
  theta/1 -> abc to dq5/2, abc to dq6/2, abc to dq1/2, abc to dq2/2, abc to dq4/2, abc to dq3/2
  abc to dq1/1 -> "Power (dq0, Instantaneous)"/2
  abc to dq2/1 -> "Power (dq0, Instantaneous)"/1
  abc to dq3/1 -> i_dq0/1
  i_abc/1 -> abc to dq3/1, abc to dq1/1
  abc to dq5/1 -> v_s_dq0/1
  v_s_abc/1 -> abc to dq5/1
  "Power (dq0, Instantaneous)"/1 -> P_abc/1
  i_s_abc/1 -> abc to dq4/1
  "Power (dq0, Instantaneous)"/2 -> Q_abc/1
  abc to dq4/1 -> i_s_dq0/1
